simulink model "configurationExampleModel"  (R2019a)
settings: Solver=VariableStepAuto  StartTime=0.0  StopTime=10.0  RelTol=1e-3
libraries: configurationExampleLibrary x2
settings Model: Creator=jnicholson  LastModifiedBy=jnicholson

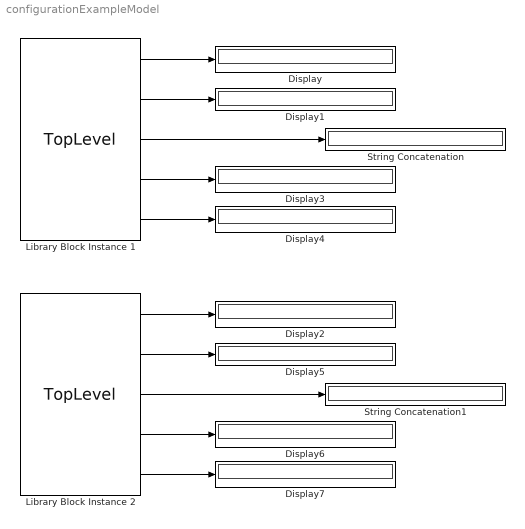
== system configurationExampleModel ==
  Display{,1..7} (8 alike) : Display
  Library Block Instance 1 : configurationExampleLibrary/TopLevel  optionA=3  optionB=2  isOptionCenabled=off  optionC=0  optionD=1  optionE=9  optionF=1
  Library Block Instance 2 : configurationExampleLibrary/TopLevel  optionA=4  optionB=1  isOptionCenabled=off  optionC=0  optionD=59  optionE=22  optionF=14
  String Concatenation : Display
  String Concatenation1 : Display
  wires:
  Library Block Instance 1/1 -> Display/1
  Library Block Instance 1/2 -> Display1/1
  Library Block Instance 1/3 -> String Concatenation/1
  Library Block Instance 1/4 -> Display3/1
  Library Block Instance 1/5 -> Display4/1
  Library Block Instance 2/5 -> Display7/1
  Library Block Instance 2/3 -> String Concatenation1/1
  Library Block Instance 2/4 -> Display6/1
  Library Block Instance 2/2 -> Display5/1
  Library Block Instance 2/1 -> Display2/1
